simulink model "ModelWithDynamics"  (R2018b)
settings: Solver=VariableStepAuto  StartTime=0.0  StopTime=10.0  RelTol=1e-3
values from neighbouring files (symbols this model uses):
  b = 0.0001    [SetConstants.m]
  J = 0.0333    [SetConstants.m]
  L = 0.3    [SetConstants.m]
settings Model: Creator=Mike  LastModifiedBy=Mike

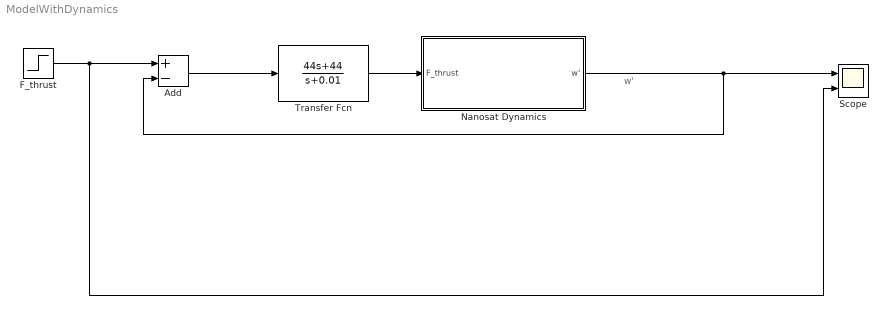
== system ModelWithDynamics ==
  note: w'
  Add : Sum  Inputs=+-
  F_thrust : Step  After=0.00184926  SampleTime=0
  Nanosat Dynamics : Subsystem
  Scope : Scope  NumInputPorts=2
  Transfer Fcn : TransferFcn  Numerator=[44 44]  Denominator=[1 0.01]
  wires:
  Nanosat Dynamics/1("w' ") -> Add/2, Scope/1
  Transfer Fcn/1 -> Nanosat Dynamics/1(F_thrust)
  Add/1 -> Transfer Fcn/1
  F_thrust/1 -> Scope/2, Add/1

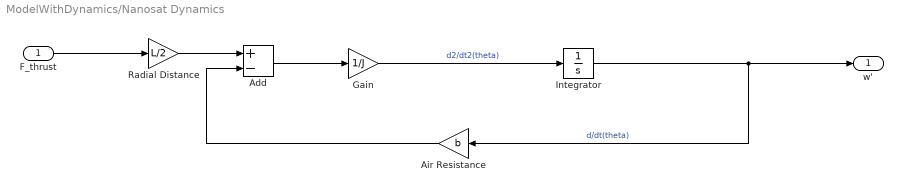
== system ModelWithDynamics/Nanosat Dynamics ==
  F_thrust : Inport
  Add : Sum  Inputs=+-
  "Air Resistance " : Gain  Gain=b
  Gain : Gain  Gain=1/J
  Integrator : Integrator
  "Radial Distance " : Gain  Gain=L/2
  "w' " : Outport
  wires:
  Add/1 -> Gain/1
  Integrator/1 -> "w' "/1, "Air Resistance "/1  "d/dt(theta)"
  Gain/1 -> Integrator/1  "d2/dt2(theta)"
  "Radial Distance "/1 -> Add/1
  F_thrust/1 -> "Radial Distance "/1
  "Air Resistance "/1 -> Add/2
